simulink model "rrrrrrr"  (R2013a)
settings: Solver=ode45  StartTime=0.0  StopTime=inf  RelTol=1e-3
undefined symbols (not defined in the file): bchgenpoly
libraries: commblkcod2 x2, commdigbbndpm3 x2, commchan3 x1, commrandsrc2 x1, commsink2 x1
settings Model: Creator=admin  LastModifiedBy=admin

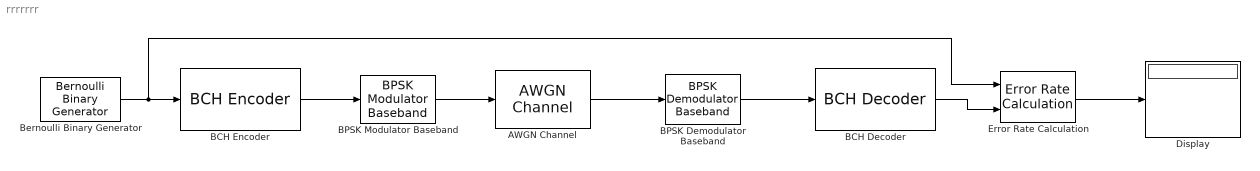
== system rrrrrrr ==
  AWGN Channel : commchan3/AWGN Channel  InputProcessing=Columns as channels (frame based)  seed=67  noiseMode="Signal to noise ratio  (Eb/No)"  EbNodB=2  EsNodB=10  SNRdB=10  bitsPerSym=1  Ps=1  Tsym=1  variance=1
  BCH Decoder : commblkcod2/BCH Decoder  n=15  k=11  specPrimPoly=off  prPoly=[1 0 0 1 1]  specGenPoly=off  genPoly=bchgenpoly(15,5)  specDisableGenCheck=off  specPuncture=off  punctVec=[ones(8,1); zeros(2,1)]  specErasurePort=off  showNumErr=off
  BCH Encoder : commblkcod2/BCH Encoder  n=15  k=11  specPrimPoly=off  prPoly=[1 0 0 1 1 ]  specGenPoly=off  genPoly=bchgenpoly(15,11)  specDisableGenCheck=off  specPuncture=off  punctVec=[ones(8,1); zeros(2,1)]
  BPSK Demodulator Baseband : commdigbbndpm3/BPSK Demodulator Baseband  Ph=0  DecType=Hard decision  VarSource=Dialog  Variance=1  outDtype=Inherit via internal rule  derotateFactorWordLen=16
  BPSK Modulator Baseband : commdigbbndpm3/BPSK Modulator Baseband  Ph=0  outDtype=double  outWordLen=16  outUDDataType=sfix(16)  outFracLenMode=Best precision  outFracLen=15
  Bernoulli Binary Generator : commrandsrc2/Bernoulli Binary Generator  P=0.5  seed=67  Ts=1  frameBased=on  sampPerFrame=11  orient=off  outDataType=double
  Display : Display
  Error Rate Calculation : commsink2/Error Rate Calculation  N=0  st_delay=0  cp_mode=Entire frame  subframe=[]  PMode=Port  WsName=ErrorVec  RsMode2=off  stop=off  numErr=100  maxBits=1e6
  wires:
  Bernoulli Binary Generator/1 -> Error Rate Calculation/1, BCH Encoder/1
  BCH Encoder/1 -> BPSK Modulator Baseband/1
  BPSK Modulator Baseband/1 -> AWGN Channel/1
  AWGN Channel/1 -> BPSK Demodulator Baseband/1
  BPSK Demodulator Baseband/1 -> BCH Decoder/1
  BCH Decoder/1 -> Error Rate Calculation/2
  Error Rate Calculation/1 -> Display/1
